simulink model "DefaultTransitiontoState_2018a"  (R2018a)
settings: Solver=VariableStepAuto  StartTime=0.0  StopTime=10.0  RelTol=1e-3
settings Model: Creator=apple  LastModifiedBy=apple
settings DataIOCC: ReturnWorkspaceOutputs=on
settings SFSimCC: SimUseLocalCustomCode=on
settings RTWCC: RTWUseLocalCustomCode=on

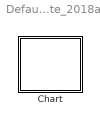
== system DefaultTransitiontoState_2018a ==
  Chart : Stateflow chart  TreatAsAtomicUnit=on

== stateflow chart DefaultTransitiontoState_2018a/Chart ==
  state A
    en:fprintf("Entry A");
    du:fprintf("During A");
    ex:fprintf("Exit A");
  state B
    en:fprintf("Entry B");
    du:fprintf("During B");
    ex:fprintf("Exit B");
    state B1
      en:fprintf("Entry B1");
      du:fprintf("During B1");
      ex:fprintf("Exit B1");
    state B2
    (default) -> B1
  (default) -> A
  A -> B : E_one/{fprintf("Transition Action");}
  events: E_one local FUNCTION_CALL_EVENT
